simulink subsystem "InertialNavigationSolution"  (R2021a)
settings: Solver=VariableStepAuto  StartTime=0.0  StopTime=10.0  RelTol=1e-3
undefined symbols (not defined in the file): q0
libraries: aerolibutil x1, sharedutil x1
settings Model: Creator=jmher  LastModifiedBy=jmher

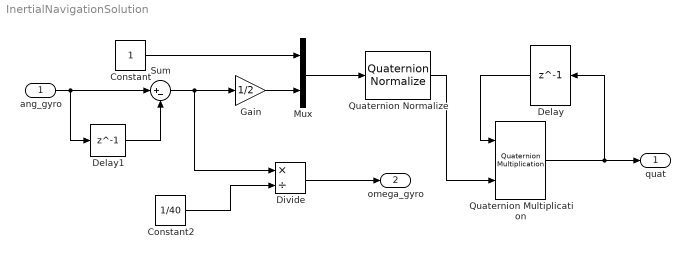
== system InertialNavigationSolution ==
  ang_gyro : Inport  SampleTime=1/40
  Constant : Constant
  Constant2 : Constant  Value=1/40
  Delay : Delay  DelayLength=1  InitialCondition=q0
  Delay1 : Delay  DelayLength=1
  Divide : Product  Inputs=*/
  Gain : Gain  Gain=1/2
  Mux : Mux  Inputs=2
  Quaternion Multiplication : aerolibutil/Quaternion Multiplication
  Quaternion Normalize : sharedutil/Quaternion Normalize  aMode=aMode
      settings: SourceProductBaseCode=AE,PW,DR,MT,UV,VE
  Sum : Sum  Inputs=|+-
  quat : Outport
  omega_gyro : Outport  Port=2
  wires:
  Gain/1 -> Mux/2
  ang_gyro/1 -> Sum/1, Delay1/1
  Constant2/1 -> Divide/2
  Constant/1 -> Mux/1
  Sum/1 -> Divide/1, Gain/1
  Quaternion Multiplication/1 -> Delay/1, quat/1
  Quaternion Normalize/1 -> Quaternion Multiplication/2
  Mux/1 -> Quaternion Normalize/1
  Divide/1 -> omega_gyro/1
  Delay1/1 -> Sum/2
  Delay/1 -> Quaternion Multiplication/1
